simulink model "Plant"  (R2018b)
settings: configuration reference "plant_config" (kept outside this file)
values from neighbouring files (symbols this model uses):
  PLANT_EXPORT = Simulink.Parameter(PLANT_EXPORT_VALUE)    [plant_model_init.m]
  PLANT_PARAM = Simulink.Parameter(PLANT_PARAM_VALUE)    [plant_model_init.m]
undefined symbols (not defined in the file or in its folder): acc_x, acc_x_O, acc_y, acc_y_O, acc_z, acc_z_O, alt, alt_0, day, DiscIntNeverNeededParam, fixType, flags, ground_force, gSpeed, gyr_x, gyr_y, gyr_z, h_R, hAcc, heading, headingAcc, height, hMSL, hour, iTOW, lat, lon, M_BO, M_OB, mag_x, mag_y, mag_z, month, nano, numSV, pDOP, phi, PLANT_CONST, plant_model, pressure, prop_vel, psi, quat, reserved1, reserved2, rot_x_B, rot_y_B, rot_z_B, sAcc, sec, Sensor_Model, tAcc, temperature, temprature, theta, timestamp, vAcc, valid, vel_x_O, vel_y_O ... (+7)
libraries: FMT_Model_Lib x22, simulink x12, dspsrcs4 x6, aerolibatmos2 x1
(part 2 of 2)

== system Plant/Sensor_Model/Sensor_MAG/Magnetometer ==
  States : Inport
  Enable_Errors : Inport  Port=2
  Bus_Constructor : Subsystem
  Physical_Model : Subsystem
  Sensor_Model : Subsystem
  Mag_Raw : Outport
  wires:
  Bus_Constructor/1(Mag_Raw) -> Mag_Raw/1
  Sensor_Model/1(y) -> Bus_Constructor/1(Output)
  States/1 -> Physical_Model/1(States)
  Physical_Model/1(mag_B_gauss) -> Sensor_Model/2(u)
  Enable_Errors/1 -> Sensor_Model/1(Enable_Errors)

== system Plant/Actuators/Motors/ESCs/Rotor_Delay ==
  in : Inport
  Discrete-Time Integrator : DiscreteIntegrator  gainval=K  SampleTime=-1  ICPrevOutput=DiscIntNeverNeededParam  ICPrevScaledInput=DiscIntNeverNeededParam
  Gain : Gain  Gain=1/T
  Subtract : Sum  Inputs=+-
  out : Outport
  wires:
  in/1 -> Subtract/1
  Subtract/1 -> Gain/1
  Gain/1 -> Discrete-Time Integrator/1
  Discrete-Time Integrator/1 -> Subtract/2, out/1

== system Plant/Actuators/Motors/ESCs/Rotor_Speed ==
  u0 : Inport
  Add : Sum
  Compare To Constant : simulink/Logic and Bit Operations/Compare To Constant  relop=>  const=0.1  OutDataTypeStr=boolean
  Constant1 : Constant  Value=p  OutDataTypeStr=single
  Gain1 : Gain  Gain=k  OutDataTypeStr=Inherit: Same as input
  Multiply : Product
  Saturation1 : Saturate  UpperLimit=9999999  LowerLimit=0
  omega_B_radPs : Outport
  wires:
  Multiply/1 -> Saturation1/1
  Gain1/1 -> Add/1
  Saturation1/1 -> omega_B_radPs/1
  u0/1 -> Compare To Constant/1, Gain1/1
  Constant1/1 -> Add/2
  Compare To Constant/1 -> Multiply/1
  Add/1 -> Multiply/2

== system Plant/Actuators/Motors/Force/Rotor_Thrust ==
  rotor_speed_radPs : Inport
  Multiply : Product  OutDataTypeStr=Inherit: Same as first input
  Square : Math  Operator=square  SaturateOnIntegerOverflow=on
  cT : Constant  Value=cT
  thrust_B_N : Outport
  wires:
  rotor_speed_radPs/1 -> Square/1
  Square/1 -> Multiply/1
  cT/1 -> Multiply/2
  Multiply/1 -> thrust_B_N/1

== system Plant/Actuators/Motors/Torque/Gyroscopic_Torque ==
  rotor_speed_radPs : Inport
  omega_B_radPs : Inport  Port=2
  Add : Sum  Inputs=--++
  Constant : Constant  Value=[0;0;Im]  OutDataTypeStr=single
  Cross Product : FMT_Model_Lib/Math/Cross Product
      settings: SourceProductName=FMT Toolbox
  Demux : Demux
  Multiply : Product
  gyroscopic_torque : Outport
  wires:
  Demux/1 -> Add/1
  Constant/1 -> Cross Product/1
  Demux/4 -> Add/4
  Add/1 -> Multiply/1
  Demux/3 -> Add/3
  Demux/2 -> Add/2
  omega_B_radPs/1 -> Multiply/2
  Multiply/1 -> Cross Product/2
  Cross Product/1 -> gyroscopic_torque/1
  rotor_speed_radPs/1 -> Demux/1

== system Plant/Actuators/Motors/Torque/Rotor_Torque ==
  rotor_speed_radPs : Inport
  Multiply : Product  Multiplication=Matrix(*)
  Square : Math  Operator=square  SaturateOnIntegerOverflow=on
  X_Frame_CM : Constant  Value=[-L*cT,L*cT,L*cT,-L*cT;L*cT,-L*cT,L*cT,-L*cT;cQ,cQ,-cQ,-cQ]  OutDataTypeStr=single
  rotor_torque : Outport
  wires:
  X_Frame_CM/1 -> Multiply/1
  Square/1 -> Multiply/2
  Multiply/1 -> rotor_torque/1
  rotor_speed_radPs/1 -> Square/1

== system Plant/Kinematic_Equation/Attitude_Dynamic/Quaternuin_Update/Quaternion_Update_Maxtrix ==
  omega_B_radPs : Inport
  Constant{,1..3} (4 alike) : Constant  Value=0  OutDataTypeStr=single
  Demux : Demux  Outputs=3
  Gain{1..4,6..7} (6 alike) : Gain  Gain=-1  OutDataTypeStr=Inherit: Same as input
  Matrix Concatenate{,1..3} (4 alike) : Concatenate  NumInputs=4
  Matrix Concatenate4 : Concatenate  NumInputs=4  Mode=Multidimensional array  ConcatenateDimension=2
  W : Outport
  wires:
  Gain1/1 -> Matrix Concatenate1/1
  Gain7/1 -> Matrix Concatenate3/2
  Matrix Concatenate2/1 -> Matrix Concatenate4/3  "col3"
  Constant2/1 -> Matrix Concatenate2/3
  Matrix Concatenate4/1 -> W/1
  Demux/1 -> Matrix Concatenate/2, Gain1/1, Gain4/1, Matrix Concatenate3/3  "w1"
  Matrix Concatenate/1 -> Matrix Concatenate4/1  "col1"
  Matrix Concatenate1/1 -> Matrix Concatenate4/2  "col2"
  Constant3/1 -> Matrix Concatenate3/4
  Gain6/1 -> Matrix Concatenate3/1
  Constant1/1 -> Matrix Concatenate1/2
  Matrix Concatenate3/1 -> Matrix Concatenate4/4  "col4"
  Demux/2 -> Matrix Concatenate1/4, Gain3/1, Gain7/1, Matrix Concatenate/3  "w2"
  Constant/1 -> Matrix Concatenate/1
  Gain3/1 -> Matrix Concatenate2/1
  Demux/3 -> Gain2/1, Matrix Concatenate2/2, Gain6/1, Matrix Concatenate/4  "w3"
  Gain2/1 -> Matrix Concatenate1/3
  omega_B_radPs/1 -> Demux/1
  Gain4/1 -> Matrix Concatenate2/4

== system Plant/Sensor_Model/Sensor_Barometer/Barometer/Physical_Model ==
  States : Inport
  Bus Selector1 : BusSelector  OutputSignals=Plant_States.alt
  Data Type Conversion : DataTypeConversion  OutDataTypeStr=single
  ISA Atmosphere Model : aerolibatmos2/ISA Atmosphere Model  custom=off  g=9.80665  gamma=1.4  R=287.0531  L=0.0065  h_trop=11000  h_strat=20000  rho0=1.225  P0=101325  T0=288.15  h0=0
      settings: SourceProductName=Aerospace Blockset
  Terminator : Terminator
  Terminator1 : Terminator
  Pressure_Pa : Outport
  Temperature_K : Outport  Port=2
  wires:
  States/1 -> Bus Selector1/1
  ISA Atmosphere Model/1 -> Temperature_K/1
  ISA Atmosphere Model/2 -> Terminator1/1
  ISA Atmosphere Model/4 -> Terminator/1
  Bus Selector1/1 -> Data Type Conversion/1  "<alt>"
  ISA Atmosphere Model/3 -> Pressure_Pa/1
  Data Type Conversion/1 -> ISA Atmosphere Model/1

== system Plant/Sensor_Model/Sensor_Barometer/Barometer/Sensor_Model ==
  Enable_Errors : Inport
  u : Inport  Port=2
  Add : Sum  InputSameDT=on  OutDataTypeStr=Inherit: Same as first input
  Saturation : Saturate  UpperLimit=Sensor_Model.Baro.Upper_limit  LowerLimit=Sensor_Model.Baro.Lower_limit  OutDataTypeStr=single
  Sensor_Error : Subsystem
  Sensor_Noise : Subsystem
  Switch : Switch  Criteria=u2 > Threshold
  y : Outport
  wires:
  Switch/1 -> y/1
  Saturation/1 -> Add/1
  Sensor_Error/1(y) -> Saturation/1
  Enable_Errors/1 -> Switch/2
  u/1 -> Switch/3, Sensor_Error/1(u)
  Add/1 -> Switch/1
  Sensor_Noise/1(noise) -> Add/2

== system Plant/Sensor_Model/Sensor_GPS/Bus_Constructor/GroundSpeed ==
  u_O_mPs : Inport
  v_O_mPs : Inport  Port=2
  Add : Sum
  Math Function : Math  Operator=square  SaturateOnIntegerOverflow=on
  Math Function1 : Math  Operator=square  SaturateOnIntegerOverflow=on
  Saturation : Saturate  UpperLimit=inf  LowerLimit=0
  Sqrt : Sqrt  SaturateOnIntegerOverflow=on
  gSpeed_mPs : Outport
  wires:
  Sqrt/1 -> gSpeed_mPs/1
  Math Function/1 -> Add/1
  Math Function1/1 -> Add/2
  Saturation/1 -> Sqrt/1
  Add/1 -> Saturation/1
  u_O_mPs/1 -> Math Function/1
  v_O_mPs/1 -> Math Function1/1

== system Plant/Sensor_Model/Sensor_GPS/Bus_Constructor/WGS84_Position ==
  pos_WGS84 : Inport
  Demux1 : Demux  Outputs=3
  Signal Conversion : SignalConversion  OverrideOpt=off
  Signal Conversion1 : SignalConversion  OverrideOpt=off
  Signal Conversion2 : SignalConversion  OverrideOpt=off
  lon : Outport
  lat : Outport  Port=2
  height : Outport  Port=3
  wires:
  Demux1/3 -> Signal Conversion2/1  "POS_h_WGS84"
  Signal Conversion/1 -> lon/1
  Demux1/1 -> Signal Conversion/1  "POS_lon_WGS84"
  pos_WGS84/1 -> Demux1/1
  Demux1/2 -> Signal Conversion1/1  "POS_lat_WGS84"
  Signal Conversion1/1 -> lat/1
  Signal Conversion2/1 -> height/1

== system Plant/Sensor_Model/Sensor_GPS/GPS/Bus_Constructor ==
  WGS84_pos_meas : Inport
  vel_O_meas : Inport  Port=2
  numSV : Inport  Port=3
  fixType : Inport  Port=4
  h_Acc_m : Inport  Port=5
  v_Acc_m : Inport  Port=6
  s_Acc_mDs : Inport  Port=7
  Bus Creator : BusCreator  Inputs=7
  GPS_Raw : Outport
  wires:
  WGS84_pos_meas/1 -> Bus Creator/1  "WGS84_pos"
  vel_O_meas/1 -> Bus Creator/2  "vel_O"
  numSV/1 -> Bus Creator/3  "numSV"
  fixType/1 -> Bus Creator/4  "fixType"
  h_Acc_m/1 -> Bus Creator/5  "hAcc"
  v_Acc_m/1 -> Bus Creator/6  "vAcc"
  s_Acc_mDs/1 -> Bus Creator/7  "sAcc"
  Bus Creator/1 -> GPS_Raw/1

== system Plant/Sensor_Model/Sensor_GPS/GPS/Physical_Model ==
  note: Transfer Delay
  States : Inport
  Bus Selector : BusSelector  OutputSignals=Plant_States.lon,Plant_States.lat,Plant_States.alt
  Bus Selector1 : BusSelector  OutputSignals=Plant_States.vel_x_O,Plant_States.vel_y_O,Plant_States.vel_z_O
  Delay : Delay  DelayLength=150/(PLANT_CONST.dt*1e3)
  Delay1 : Delay  DelayLength=100/(PLANT_CONST.dt*1e3)
  Vector Concatenate : Concatenate  NumInputs=3  Mode=Multidimensional array
  Vector Concatenate1 : Concatenate  NumInputs=3  Mode=Multidimensional array
  WGS84_pos_rad : Outport  Unit=rad/s
  vel_O_mPs : Outport  Port=2  Unit=m/s  PortDimensions=[3 1]
  wires:
  Bus Selector/3 -> Vector Concatenate/3  "<alt>"
  Bus Selector/2 -> Vector Concatenate/2  "<lat>"
  Bus Selector/1 -> Vector Concatenate/1  "<lon>"
  Vector Concatenate/1 -> Delay/1
  Bus Selector1/2 -> Vector Concatenate1/2  "<vel_y_O>"
  Bus Selector1/3 -> Vector Concatenate1/3  "<vel_z_O>"
  States/1 -> Bus Selector1/1, Bus Selector/1
  Vector Concatenate1/1 -> Delay1/1
  Bus Selector1/1 -> Vector Concatenate1/1  "<vel_x_O>"
  Delay/1 -> WGS84_pos_rad/1
  Delay1/1 -> vel_O_mPs/1

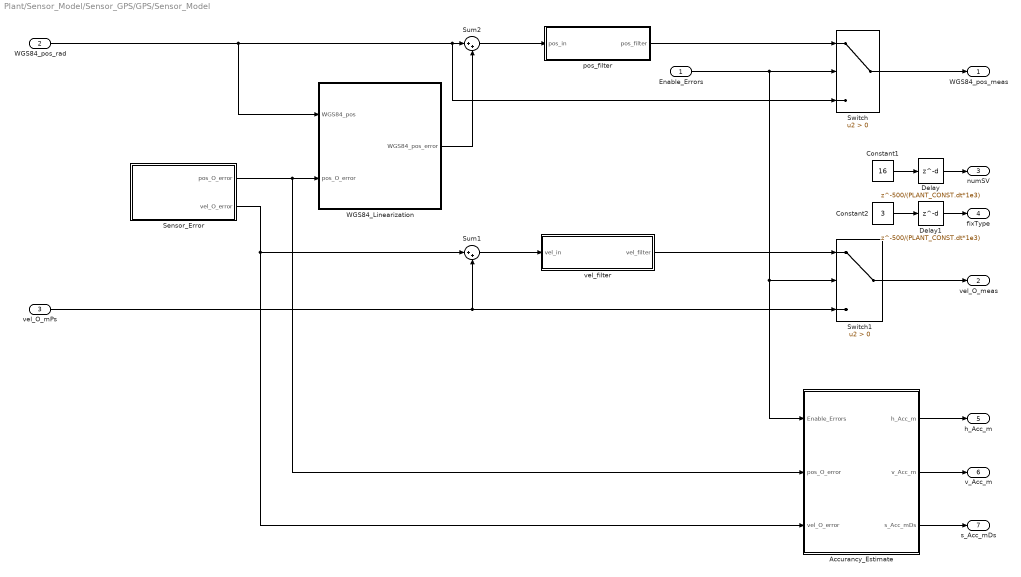
== system Plant/Sensor_Model/Sensor_GPS/GPS/Sensor_Model ==
  Enable_Errors : Inport
  WGS84_pos_rad : Inport  Port=2
  vel_O_mPs : Inport  Port=3
  Accurancy_Estimate : Subsystem
  Constant1 : Constant  Value=16  OutDataTypeStr=Inherit: Inherit via back propagation
  Constant2 : Constant  Value=3  OutDataTypeStr=Inherit: Inherit via back propagation
  Delay : Delay  DelayLength=500/(PLANT_CONST.dt*1e3)
  Delay1 : Delay  DelayLength=500/(PLANT_CONST.dt*1e3)
  Sensor_Error : Subsystem
  Sum1 : Sum  Inputs=|++
  Sum2 : Sum  Inputs=|++
  Switch : Switch  Criteria=u2 > Threshold
  Switch1 : Switch  Criteria=u2 > Threshold
  WGS84_Linearization : Subsystem
  pos_filter : Subsystem
  vel_filter : Subsystem
  WGS84_pos_meas : Outport
  vel_O_meas : Outport  Port=2
  numSV : Outport  Port=3
  fixType : Outport  Port=4
  h_Acc_m : Outport  Port=5
  v_Acc_m : Outport  Port=6
  s_Acc_mDs : Outport  Port=7
  wires:
  Constant2/1 -> Delay1/1
  Constant1/1 -> Delay/1
  Switch/1 -> WGS84_pos_meas/1
  Switch1/1 -> vel_O_meas/1
  Sum2/1 -> pos_filter/1(pos_in)
  Sensor_Error/1(pos_O_error) -> Accurancy_Estimate/2(pos_O_error), WGS84_Linearization/2(pos_O_error)
  Sum1/1 -> vel_filter/1(vel_in)
  Sensor_Error/2(vel_O_error) -> Accurancy_Estimate/3(vel_O_error), Sum1/1
  WGS84_Linearization/1(WGS84_pos_error) -> Sum2/2
  Accurancy_Estimate/1(h_Acc_m) -> h_Acc_m/1
  Accurancy_Estimate/3(s_Acc_mDs) -> s_Acc_mDs/1
  Accurancy_Estimate/2(v_Acc_m) -> v_Acc_m/1
  pos_filter/1(pos_filter) -> Switch/1
  WGS84_pos_rad/1 -> Switch/3, Sum2/1, WGS84_Linearization/1(WGS84_pos)
  vel_O_mPs/1 -> Switch1/3, Sum1/2
  vel_filter/1(vel_filter) -> Switch1/1
  Enable_Errors/1 -> Switch/2, Accurancy_Estimate/1(Enable_Errors), Switch1/2
  Delay/1 -> numSV/1
  Delay1/1 -> fixType/1

== system Plant/Sensor_Model/Sensor_IMU/Accelerometer/Bus_Constructor ==
  Output : Inport
  Bus Creator : BusCreator  Inputs=3
  Demux : Demux  Outputs=3
  Acc_Raw : Outport
  wires:
  Demux/2 -> Bus Creator/2  "Acc_y_mPs2"
  Demux/3 -> Bus Creator/3  "Acc_z_mPs2"
  Demux/1 -> Bus Creator/1  "Acc_x_mPs2"
  Bus Creator/1 -> Acc_Raw/1
  Output/1 -> Demux/1

== system Plant/Sensor_Model/Sensor_IMU/Accelerometer/Physical_Model ==
  States : Inport
  Enable_Errors : Inport  Port=2
  Sum : Sum  Inputs=|++
  Switch : Switch  Criteria=u2 > Threshold  OutDataTypeStr=single
  Vibration_Model : Subsystem  TreatAsAtomicUnit=on  mask{gain=Sensor_Model.Acc.Vibration.Gain}
      mask prompts: gain "Vibration gain"
      mask help: propeller vibration model
      settings: RTWSystemCode=Inline
  prop_vel : Subsystem
  specific_force : Subsystem
  sfor_B_mPs2 : Outport  Unit=m/s^2
  wires:
  States/1 -> specific_force/1(States), prop_vel/1(States)
  Switch/1 -> sfor_B_mPs2/1
  prop_vel/1(omega_radDs) -> Vibration_Model/1(prop_rot_radPs)
  specific_force/1(sfor_B_mPs2) -> Sum/2, Switch/3
  Enable_Errors/1 -> Switch/2
  Vibration_Model/1(vibration) -> Sum/1
  Sum/1 -> Switch/1

== system Plant/Sensor_Model/Sensor_IMU/Accelerometer/Sensor_Model ==
  Enable_Errors : Inport
  u : Inport  Port=2
  First Order LPF : FMT_Model_Lib/Filter/First Order LPF  fc=Sensor_Model.Acc.Cutoff_frequency_Hz
      settings: SourceProductName=FMT Toolbox
  Saturation : Saturate  UpperLimit=Sensor_Model.Acc.Upper_limit  LowerLimit=Sensor_Model.Acc.Lower_limit
  Sensor_Error : Subsystem
  Sensor_Noise : Subsystem
  Sum : Sum  Inputs=|++
  Switch : Switch  Criteria=u2 > Threshold
  y : Outport
  wires:
  Switch/1 -> y/1
  Saturation/1 -> Sum/1
  First Order LPF/1 -> Saturation/1
  Sensor_Error/1(y) -> First Order LPF/1
  Sensor_Noise/1(noise) -> Sum/2
  Enable_Errors/1 -> Switch/2
  u/1 -> Switch/3, Sensor_Error/1(u)
  Sum/1 -> Switch/1

== system Plant/Sensor_Model/Sensor_IMU/Gyroscope/Bus_Constructor ==
  Output : Inport
  Bus Creator : BusCreator  Inputs=3
  Demux : Demux  Outputs=3
  Gyro_Raw : Outport
  wires:
  Demux/1 -> Bus Creator/1  "Gyro_x_radPs"
  Demux/2 -> Bus Creator/2  "Gyro_y_radPs"
  Demux/3 -> Bus Creator/3  "Gyro_z_radPs"
  Bus Creator/1 -> Gyro_Raw/1
  Output/1 -> Demux/1

== system Plant/Sensor_Model/Sensor_IMU/Gyroscope/Physical_Model ==
  States : Inport
  Enable_Errors : Inport  Port=2
  Sum : Sum  Inputs=|++
  Switch : Switch  Criteria=u2 > Threshold
  Vibration_Model : Subsystem  TreatAsAtomicUnit=on  mask{gain=Sensor_Model.Gyro.Vibration.Gain}
      mask prompts: gain "Vibration gain"
      mask help: propeller vibration model
      settings: RTWSystemCode=Inline
  prop_vel : Subsystem
  rotation_speed : Subsystem
  gyr_B_radDs : Outport  Unit=rad/s
  wires:
  States/1 -> rotation_speed/1(States), prop_vel/1(States)
  Switch/1 -> gyr_B_radDs/1
  prop_vel/1(omega_radPs) -> Vibration_Model/1(prop_rot_radPs)
  rotation_speed/1(rot_radPs) -> Sum/2, Switch/3
  Enable_Errors/1 -> Switch/2
  Vibration_Model/1(vibration) -> Sum/1
  Sum/1 -> Switch/1

== system Plant/Sensor_Model/Sensor_IMU/Gyroscope/Sensor_Model ==
  Enable_Errors : Inport
  u : Inport  Port=2
  First Order LPF : FMT_Model_Lib/Filter/First Order LPF  fc=Sensor_Model.Gyro.Cutoff_frequency_Hz
      settings: SourceProductName=FMT Toolbox
  Saturation : Saturate  UpperLimit=Sensor_Model.Gyro.Range  LowerLimit=-Sensor_Model.Gyro.Range
  Sensor_Error : Subsystem
  Sensor_Noise : Subsystem
  Sum : Sum  Inputs=|++
  Switch : Switch  Criteria=u2 > Threshold
  y : Outport
  wires:
  Switch/1 -> y/1
  Saturation/1 -> Sum/1
  First Order LPF/1 -> Saturation/1
  Sensor_Error/1(y) -> First Order LPF/1
  Sensor_Noise/1(noise) -> Sum/2
  Enable_Errors/1 -> Switch/2
  u/1 -> Switch/3, Sensor_Error/1(u)
  Sum/1 -> Switch/1

== system Plant/Sensor_Model/Sensor_MAG/Magnetometer/Bus_Constructor ==
  Output : Inport
  Bus Creator : BusCreator  Inputs=3
  Demux : Demux  Outputs=3
  Mag_Raw : Outport
  wires:
  Demux/2 -> Bus Creator/2  "Mag_y_gauss"
  Demux/1 -> Bus Creator/1  "Mag_x_gauss"
  Bus Creator/1 -> Mag_Raw/1
  Demux/3 -> Bus Creator/3  "Mag_z_gauss"
  Output/1 -> Demux/1

== system Plant/Sensor_Model/Sensor_MAG/Magnetometer/Physical_Model ==
  States : Inport
  Bus Selector : BusSelector  OutputSignals=Plant_States.lat,Plant_States.lon
  Bus Selector1 : BusSelector  OutputSignals=Extended_States.M_BO
  Product : Product  Multiplication=Matrix(*)  RndMeth=Zero  InputSameDT=on  OutDataTypeStr=Inherit: Same as first input
  WMM_LUT : Subsystem  mask{wmm_magnitude=Sensor_Model.Mag.WMM_Mag, wmm_declination=Sensor_Model.Mag.WMM_Dec, wmm_inclination=Sensor_Model.Mag.WMM_Inc, resolution=10}
      mask prompts: wmm_magnitude "WMM Magnitude Lookup Table"; wmm_declination "WMM Declination Lookup Table"; wmm_inclination "WMM Inclination Lookup Table"; resolution "Resolution (deg)"
  magnetic_field : Subsystem
  mag_B_gauss : Outport  Unit=T  PortDimensions=[3 1]
  wires:
  States/1 -> Bus Selector1/1, Bus Selector/1
  Bus Selector/2 -> WMM_LUT/2(lon_rad)  "<lon>"
  Bus Selector/1 -> WMM_LUT/1(lat_rad)  "<lat>"
  Bus Selector1/1 -> Product/1  "<M_BO>"
  Product/1 -> mag_B_gauss/1
  magnetic_field/1(mag_O_gauss) -> Product/2
  WMM_LUT/1(magnitude_uT) -> magnetic_field/1(magnitude_uT)
  WMM_LUT/2(declination_deg) -> magnetic_field/2(declination_deg)
  WMM_LUT/3(inclination_deg) -> magnetic_field/3(inclination_deg)

== system Plant/Sensor_Model/Sensor_MAG/Magnetometer/Sensor_Model ==
  Enable_Errors : Inport
  u : Inport  Port=2
  Add : Sum  InputSameDT=on  OutDataTypeStr=Inherit: Same as first input
  Saturation : Saturate  UpperLimit=Sensor_Model.Mag.Upper_limit  LowerLimit=Sensor_Model.Mag.Lower_limit
  Sensor_Error : Subsystem
  Sensor_Noise : Subsystem
  Switch : Switch  Criteria=u2 > Threshold
  y : Outport
  wires:
  Switch/1 -> y/1
  Saturation/1 -> Add/1
  Sensor_Error/1(y) -> Saturation/1
  Sensor_Noise/1(noise) -> Add/2
  Enable_Errors/1 -> Switch/2
  u/1 -> Switch/3, Sensor_Error/1(u)
  Add/1 -> Switch/1

== system Plant/Sensor_Model/Sensor_Barometer/Barometer/Sensor_Model/Sensor_Error ==
  u : Inport
  Constant3 : Constant  Value=Sensor_Model.Baro.Bias  VectorParams1D=off  OutDataTypeStr=single
  Sum : Sum  Inputs=|++  InputSameDT=on  OutDataTypeStr=Inherit: Same as first input
  y : Outport
  wires:
  Sum/1 -> y/1
  u/1 -> Sum/1
  Constant3/1 -> Sum/2

== system Plant/Sensor_Model/Sensor_Barometer/Barometer/Sensor_Model/Sensor_Noise ==
  Random Source : dspsrcs4/Random Source  SrcType=Gaussian  NormMethod=Ziggurat  CltLength=12  MinVal=0  MaxVal=1  MeanVal=0  VarVal=Sensor_Model.Baro.Variance  RepMode=Repeatable  rawSeed=1  IsInherit=off  SampMode=Discrete  SampTime=-1  SampFrame=1  DataType=Single  OutComplex=Real  OutputFrames=off
  noise : Outport
  wires:
  Random Source/1 -> noise/1

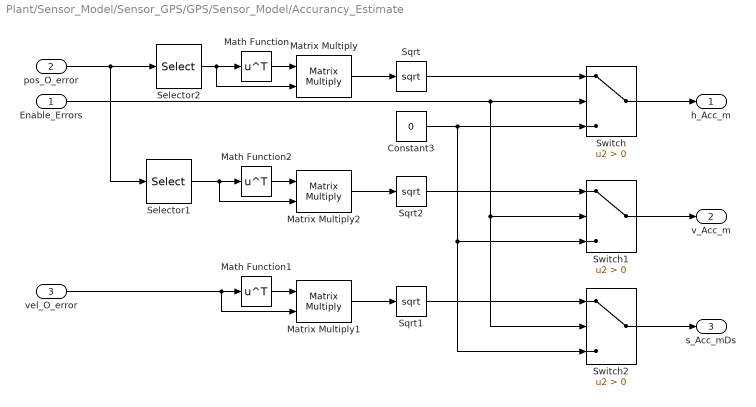
== system Plant/Sensor_Model/Sensor_GPS/GPS/Sensor_Model/Accurancy_Estimate ==
  Enable_Errors : Inport
  pos_O_error : Inport  Port=2
  vel_O_error : Inport  Port=3
  Constant3 : Constant  Value=0
  Math Function : Math  Operator=transpose  SaturateOnIntegerOverflow=on
  Math Function1 : Math  Operator=transpose  SaturateOnIntegerOverflow=on
  Math Function2 : Math  Operator=transpose  SaturateOnIntegerOverflow=on
  Matrix Multiply : Product  Multiplication=Matrix(*)
  Matrix Multiply1 : Product  Multiplication=Matrix(*)
  Matrix Multiply2 : Product  Multiplication=Matrix(*)
  Selector1 : Selector  InputPortWidth=3  IndexOptions=Index vector (dialog)  Indices=3  OutputSizes=1
  Selector2 : Selector  InputPortWidth=3  IndexOptions=Index vector (dialog)  Indices=[1 2]  OutputSizes=1
  Sqrt : Sqrt  OutputSignalType=real  SaturateOnIntegerOverflow=on
  Sqrt1 : Sqrt  OutputSignalType=real  SaturateOnIntegerOverflow=on
  Sqrt2 : Sqrt  OutputSignalType=real  SaturateOnIntegerOverflow=on
  Switch : Switch  Criteria=u2 > Threshold
  Switch1 : Switch  Criteria=u2 > Threshold
  Switch2 : Switch  Criteria=u2 > Threshold
  h_Acc_m : Outport
  v_Acc_m : Outport  Port=2
  s_Acc_mDs : Outport  Port=3
  wires:
  Switch/1 -> h_Acc_m/1
  pos_O_error/1 -> Selector1/1, Selector2/1
  Switch1/1 -> v_Acc_m/1
  Selector1/1 -> Math Function2/1, Matrix Multiply2/2
  Switch2/1 -> s_Acc_mDs/1
  Math Function1/1 -> Matrix Multiply1/1
  Math Function2/1 -> Matrix Multiply2/1
  Math Function/1 -> Matrix Multiply/1
  Selector2/1 -> Matrix Multiply/2, Math Function/1
  Matrix Multiply1/1 -> Sqrt1/1
  Matrix Multiply/1 -> Sqrt/1
  Matrix Multiply2/1 -> Sqrt2/1
  vel_O_error/1 -> Matrix Multiply1/2, Math Function1/1
  Sqrt/1 -> Switch/1
  Sqrt2/1 -> Switch1/1
  Enable_Errors/1 -> Switch2/2, Switch1/2, Switch/2
  Sqrt1/1 -> Switch2/1
  Constant3/1 -> Switch2/3, Switch1/3, Switch/3

== system Plant/Sensor_Model/Sensor_GPS/GPS/Sensor_Model/Sensor_Error ==
  Random Source : dspsrcs4/Random Source  SrcType=Gaussian  NormMethod=Ziggurat  CltLength=12  MinVal=0  MaxVal=1  MeanVal=0  VarVal=[0.2;0.2;0.4].^2  RepMode=Repeatable  rawSeed=1  IsInherit=off  SampMode=Discrete  SampTime=-1  SampFrame=1  DataType=Single  OutComplex=Real  OutputFrames=off
  Random Source1 : dspsrcs4/Random Source  SrcType=Gaussian  NormMethod=Ziggurat  CltLength=12  MinVal=0  MaxVal=1  MeanVal=0  VarVal=[0.01;0.01;0.01].^2  RepMode=Repeatable  rawSeed=1  IsInherit=off  SampMode=Discrete  SampTime=-1  SampFrame=1  DataType=Single  OutComplex=Real  OutputFrames=off
  pos_O_error : Outport
  vel_O_error : Outport  Port=2
  wires:
  Random Source/1 -> pos_O_error/1
  Random Source1/1 -> vel_O_error/1

== system Plant/Sensor_Model/Sensor_GPS/GPS/Sensor_Model/WGS84_Linearization ==
  WGS84_pos : Inport
  pos_O_error : Inport  Port=2
  Demux2 : Demux  Outputs=3
  Divide2 : Product  Inputs=/*
  LAT2FLAT Curve : FMT_Model_Lib/Transformation/LAT2FLAT Curve
      settings: SourceProductName=FMT Toolbox
  Terminator1 : Terminator
  Terminator2 : Terminator
  Vector Concatenate2 : Concatenate  NumInputs=3  Mode=Multidimensional array
  constant1 : Constant  Value=-1
  WGS84_pos_error : Outport
  wires:
  WGS84_pos/1 -> Demux2/1
  Demux2/1 -> LAT2FLAT Curve/1
  LAT2FLAT Curve/2 -> Vector Concatenate2/2
  pos_O_error/1 -> Divide2/2
  Vector Concatenate2/1 -> Divide2/1
  LAT2FLAT Curve/1 -> Vector Concatenate2/1
  Demux2/2 -> Terminator2/1
  Demux2/3 -> Terminator1/1
  constant1/1 -> Vector Concatenate2/3
  Divide2/1 -> WGS84_pos_error/1

== system Plant/Sensor_Model/Sensor_GPS/GPS/Sensor_Model/pos_filter ==
  pos_in : Inport
  Discrete FIR Filter : DiscreteFir
  pos_filter : Outport
  wires:
  Discrete FIR Filter/1 -> pos_filter/1
  pos_in/1 -> Discrete FIR Filter/1

== system Plant/Sensor_Model/Sensor_GPS/GPS/Sensor_Model/vel_filter ==
  vel_in : Inport
  Discrete FIR Filter : DiscreteFir
  vel_filter : Outport
  wires:
  Discrete FIR Filter/1 -> vel_filter/1
  vel_in/1 -> Discrete FIR Filter/1

== system Plant/Sensor_Model/Sensor_IMU/Accelerometer/Physical_Model/Vibration_Model ==
  prop_rot_radPs : Inport  PortDimensions=[4,1]
  Compare To Constant1 : simulink/Logic and Bit Operations/Compare To Constant  relop=>  const=4*pi  OutDataTypeStr=boolean
  Discrete-Time Integrator : DiscreteIntegrator  InitialCondition=zeros(4,1)  SampleTime=-1  ICPrevOutput=DiscIntNeverNeededParam  ICPrevScaledInput=DiscIntNeverNeededParam
  Divide : Product  Inputs=*/
  Gain2 : Gain  Gain=0.5
  Gain4 : Gain  Gain=gain
  Product1 : Product  RndMeth=Zero
  Product2 : Product  RndMeth=Zero
  Reshape : Reshape  OutputDimensionality=Column vector (2-D)
  Saturation : Saturate  UpperLimit=8  LowerLimit=4
  Sum : Sum  Inputs=++|
  Sum of Elements : Sum  Inputs=+
  Sum of Elements1 : Sum  Inputs=+
  Sum of Elements2 : Sum  Inputs=+  CollapseMode=Specified dimension
  Trigonometric Function1 : Trigonometry  Operator=cos
  Trigonometric Function2 : Trigonometry
  Vector Concatenate : Concatenate  NumInputs=3  Mode=Multidimensional array
  vib_frequency : Subsystem
  vibration : Outport
  wires:
  Sum of Elements2/1 -> Saturation/1
  Saturation/1 -> Divide/2
  Divide/1 -> Gain4/1
  Compare To Constant1/1 -> Sum of Elements2/1
  Vector Concatenate/1 -> Divide/1
  Trigonometric Function1/1 -> Product1/1
  Trigonometric Function2/1 -> Product2/1
  Gain2/1 -> Vector Concatenate/3
  Sum/1 -> Gain2/1
  Sum of Elements1/1 -> Sum/2, Vector Concatenate/2
  Discrete-Time Integrator/1 -> Trigonometric Function1/1, Trigonometric Function2/1
  Sum of Elements/1 -> Vector Concatenate/1, Sum/1
  Reshape/1 -> vibration/1
  Gain4/1 -> Reshape/1
  prop_rot_radPs/1 -> Compare To Constant1/1, Discrete-Time Integrator/1, vib_frequency/1(prop_rot_radPs)
  vib_frequency/1(y) -> Product2/2, Product1/2
  Product2/1 -> Sum of Elements/1
  Product1/1 -> Sum of Elements1/1

== system Plant/Sensor_Model/Sensor_IMU/Accelerometer/Physical_Model/prop_vel ==
  States : Inport
  Bus Selector2 : BusSelector  OutputSignals=Extended_States.prop_vel
  Selector : Selector  InputPortWidth=8  IndexOptions=Index vector (dialog)  Indices=[1:4]  OutputSizes=1
  omega_radDs : Outport
  wires:
  States/1 -> Bus Selector2/1
  Bus Selector2/1 -> Selector/1  "<prop_vel>"
  Selector/1 -> omega_radDs/1

== system Plant/Sensor_Model/Sensor_IMU/Accelerometer/Physical_Model/specific_force ==
  States : Inport
  Bus Selector : BusSelector  OutputSignals=Plant_States.acc_x_O,Plant_States.acc_y_O,Plant_States.acc_z_O
  Bus Selector1 : BusSelector  OutputSignals=Extended_States.M_BO
  Gravity : Constant  Value=[0;0;Sensor_Model.g]  OutDataTypeStr=single
  Product1 : Product  Multiplication=Matrix(*)  RndMeth=Zero  InputSameDT=on  OutDataTypeStr=Inherit: Same as first input
  Sum : Sum  Inputs=|+-  InputSameDT=on  OutDataTypeStr=Inherit: Same as first input
  Vector Concatenate1 : Concatenate  NumInputs=3  Mode=Multidimensional array
  sfor_B_mPs2 : Outport  Unit=m/s^2
  wires:
  States/1 -> Bus Selector1/1, Bus Selector/1
  Bus Selector/1 -> Vector Concatenate1/1  "<acc_x_O>"
  Bus Selector/2 -> Vector Concatenate1/2  "<acc_y_O>"
  Bus Selector/3 -> Vector Concatenate1/3  "<acc_z_O>"
  Product1/1 -> sfor_B_mPs2/1
  Bus Selector1/1 -> Product1/1  "<M_BO>"
  Vector Concatenate1/1 -> Sum/1
  Sum/1 -> Product1/2
  Gravity/1 -> Sum/2

== system Plant/Sensor_Model/Sensor_IMU/Accelerometer/Sensor_Model/Sensor_Error ==
  u : Inport
  Add : Sum  InputSameDT=on  OutDataTypeStr=Inherit: Same as first input
  Constant : Constant  Value=eye(3)  OutDataTypeStr=single
  Constant1 : Constant  Value=Sensor_Model.Acc.Scalefactor_Error  VectorParams1D=off  OutDataTypeStr=single
  Constant3 : Constant  Value=Sensor_Model.Acc.Bias  VectorParams1D=off  OutDataTypeStr=single
  Product : Product  Multiplication=Matrix(*)  RndMeth=Zero  InputSameDT=on  OutDataTypeStr=Inherit: Same as first input
  Sum : Sum  Inputs=|++  InputSameDT=on  OutDataTypeStr=Inherit: Same as first input
  y : Outport
  wires:
  Sum/1 -> y/1
  Add/1 -> Product/1
  u/1 -> Product/2
  Constant1/1 -> Add/2
  Constant/1 -> Add/1
  Product/1 -> Sum/1
  Constant3/1 -> Sum/2

== system Plant/Sensor_Model/Sensor_IMU/Accelerometer/Sensor_Model/Sensor_Noise ==
  Random Source : dspsrcs4/Random Source  SrcType=Gaussian  NormMethod=Ziggurat  CltLength=12  MinVal=0  MaxVal=1  MeanVal=0  VarVal=Sensor_Model.Acc.Variance  RepMode=Repeatable  rawSeed=1  IsInherit=off  SampMode=Discrete  SampTime=-1  SampFrame=1  DataType=Single  OutComplex=Real  OutputFrames=off
  noise : Outport
  wires:
  Random Source/1 -> noise/1

== system Plant/Sensor_Model/Sensor_IMU/Gyroscope/Physical_Model/Vibration_Model ==
  prop_rot_radPs : Inport  PortDimensions=[4,1]
  Compare To Constant1 : simulink/Logic and Bit Operations/Compare To Constant  relop=>  const=4*pi  OutDataTypeStr=boolean
  Discrete-Time Integrator : DiscreteIntegrator  InitialCondition=zeros(4,1)  SampleTime=-1  ICPrevOutput=DiscIntNeverNeededParam  ICPrevScaledInput=DiscIntNeverNeededParam
  Divide : Product  Inputs=*/
  Gain2 : Gain  Gain=0.5
  Gain4 : Gain  Gain=gain
  Product1 : Product  RndMeth=Zero
  Product2 : Product  RndMeth=Zero
  Reshape : Reshape  OutputDimensionality=Column vector (2-D)
  Saturation : Saturate  UpperLimit=8  LowerLimit=4
  Sum : Sum  Inputs=++|
  Sum of Elements : Sum  Inputs=+
  Sum of Elements1 : Sum  Inputs=+
  Sum of Elements2 : Sum  Inputs=+  CollapseMode=Specified dimension
  Trigonometric Function1 : Trigonometry  Operator=cos
  Trigonometric Function2 : Trigonometry
  Vector Concatenate : Concatenate  NumInputs=3  Mode=Multidimensional array
  vib_frequency : Subsystem
  vibration : Outport
  wires:
  Sum of Elements2/1 -> Saturation/1
  Saturation/1 -> Divide/2
  Divide/1 -> Gain4/1
  Compare To Constant1/1 -> Sum of Elements2/1
  Vector Concatenate/1 -> Divide/1
  Trigonometric Function1/1 -> Product1/1
  Trigonometric Function2/1 -> Product2/1
  Gain2/1 -> Vector Concatenate/3
  Sum/1 -> Gain2/1
  Sum of Elements1/1 -> Sum/2, Vector Concatenate/2
  Discrete-Time Integrator/1 -> Trigonometric Function1/1, Trigonometric Function2/1
  Sum of Elements/1 -> Vector Concatenate/1, Sum/1
  Reshape/1 -> vibration/1
  Gain4/1 -> Reshape/1
  prop_rot_radPs/1 -> Compare To Constant1/1, Discrete-Time Integrator/1, vib_frequency/1(prop_rot_radPs)
  vib_frequency/1(y) -> Product2/2, Product1/2
  Product2/1 -> Sum of Elements/1
  Product1/1 -> Sum of Elements1/1

== system Plant/Sensor_Model/Sensor_IMU/Gyroscope/Physical_Model/prop_vel ==
  States : Inport
  Bus Selector2 : BusSelector  OutputSignals=Extended_States.prop_vel
  Selector : Selector  InputPortWidth=8  IndexOptions=Index vector (dialog)  Indices=[1:4]  OutputSizes=1
  omega_radPs : Outport
  wires:
  Selector/1 -> omega_radPs/1
  States/1 -> Bus Selector2/1
  Bus Selector2/1 -> Selector/1  "<prop_vel>"

== system Plant/Sensor_Model/Sensor_IMU/Gyroscope/Physical_Model/rotation_speed ==
  States : Inport
  Bus Selector2 : BusSelector  OutputSignals=Plant_States.rot_x_B,Plant_States.rot_y_B,Plant_States.rot_z_B
  Vector Concatenate : Concatenate  NumInputs=3  Mode=Multidimensional array
  rot_radPs : Outport
  wires:
  Vector Concatenate/1 -> rot_radPs/1
  Bus Selector2/3 -> Vector Concatenate/3  "<rot_z_B>"
  Bus Selector2/1 -> Vector Concatenate/1  "<rot_x_B>"
  Bus Selector2/2 -> Vector Concatenate/2  "<rot_y_B>"
  States/1 -> Bus Selector2/1

== system Plant/Sensor_Model/Sensor_IMU/Gyroscope/Sensor_Model/Sensor_Error ==
  u : Inport
  Add : Sum  InputSameDT=on  OutDataTypeStr=Inherit: Same as first input
  Constant1 : Constant  Value=Sensor_Model.Gyro.Scalefactor_Error  VectorParams1D=off  OutDataTypeStr=single
  Constant2 : Constant  Value=eye(3)  OutDataTypeStr=single
  Constant3 : Constant  Value=Sensor_Model.Gyro.Bias  VectorParams1D=off  OutDataTypeStr=single
  Product : Product  Multiplication=Matrix(*)  RndMeth=Zero  InputSameDT=on  OutDataTypeStr=Inherit: Same as first input
  Sum : Sum  Inputs=|++  InputSameDT=on  OutDataTypeStr=Inherit: Same as first input
  y : Outport
  wires:
  Sum/1 -> y/1
  Product/1 -> Sum/1
  u/1 -> Product/2
  Add/1 -> Product/1
  Constant1/1 -> Add/2
  Constant2/1 -> Add/1
  Constant3/1 -> Sum/2

== system Plant/Sensor_Model/Sensor_IMU/Gyroscope/Sensor_Model/Sensor_Noise ==
  Random Source : dspsrcs4/Random Source  SrcType=Gaussian  NormMethod=Ziggurat  CltLength=12  MinVal=0  MaxVal=1  MeanVal=0  VarVal=Sensor_Model.Gyro.Variance  RepMode=Repeatable  rawSeed=1  IsInherit=off  SampMode=Discrete  SampTime=-1  SampFrame=1  DataType=Single  OutComplex=Real  OutputFrames=off
  noise : Outport
  wires:
  Random Source/1 -> noise/1

== system Plant/Sensor_Model/Sensor_MAG/Magnetometer/Physical_Model/WMM_LUT ==
  lat_rad : Inport
  lon_rad : Inport  Port=2
  Add : Sum
  Declination_Lookup_Table : LookupNDDirect  Table=wmm_declination  DiagnosticForOutOfRangeInput=Error
  Demux : Demux  Outputs=2
  Inclination_Lookup_Table : LookupNDDirect  Table=wmm_inclination  DiagnosticForOutOfRangeInput=Error
  Magnitude_Lookup_Table : LookupNDDirect  Table=wmm_magnitude  DiagnosticForOutOfRangeInput=Error
  Mux : Mux  Inputs=2
  Saturation1 : Saturate  UpperLimit=size(wmm_magnitude)-1  LowerLimit=0
  offset : Constant  Value=(size(wmm_magnitude)-1)/2  OutDataTypeStr=int32
  rad_to_index : Gain  Gain=180/pi/resolution  OutDataTypeStr=int32
  magnitude_uT : Outport
  declination_deg : Outport  Port=2
  inclination_deg : Outport  Port=3
  wires:
  Inclination_Lookup_Table/1 -> inclination_deg/1
  Declination_Lookup_Table/1 -> declination_deg/1
  Magnitude_Lookup_Table/1 -> magnitude_uT/1
  offset/1 -> Add/2
  Add/1 -> Saturation1/1
  rad_to_index/1 -> Add/1
  lat_rad/1 -> Mux/1
  lon_rad/1 -> Mux/2
  Mux/1 -> rad_to_index/1
  Saturation1/1 -> Demux/1
  Demux/1 -> Magnitude_Lookup_Table/1, Inclination_Lookup_Table/1, Declination_Lookup_Table/1
  Demux/2 -> Inclination_Lookup_Table/2, Magnitude_Lookup_Table/2, Declination_Lookup_Table/2

== system Plant/Sensor_Model/Sensor_MAG/Magnetometer/Physical_Model/magnetic_field ==
  magnitude_uT : Inport
  declination_deg : Inport  Port=2
  inclination_deg : Inport  Port=3
  Constant : Constant  Value=[1;0;0]  OutDataTypeStr=single
  Gain : Gain  Gain=-pi/180
  Gain1 : Gain  Gain=pi/180
  Multiply : Product
  Multiply1 : Product  Multiplication=Matrix(*)
  Multiply2 : Product  Multiplication=Matrix(*)
  Rotation Matrix Y : FMT_Model_Lib/Transformation/Rotation Matrix Y
      settings: SourceProductName=FMT Toolbox
  Rotation Matrix Z : FMT_Model_Lib/Transformation/Rotation Matrix Z
      settings: SourceProductName=FMT Toolbox
  toGauss : Gain  Gain=0.01
  mag_O_gauss : Outport
  wires:
  Constant/1 -> Multiply/2
  Multiply/1 -> Multiply1/2  "mag_field"
  Rotation Matrix Y/1 -> Multiply1/1
  inclination_deg/1 -> Gain/1
  Gain/1 -> Rotation Matrix Y/1
  declination_deg/1 -> Gain1/1
  Gain1/1 -> Rotation Matrix Z/1
  Rotation Matrix Z/1 -> Multiply2/1
  magnitude_uT/1 -> toGauss/1
  toGauss/1 -> Multiply/1  "magnitude_gauss"
  Multiply1/1 -> Multiply2/2
  Multiply2/1 -> mag_O_gauss/1

== system Plant/Sensor_Model/Sensor_MAG/Magnetometer/Sensor_Model/Sensor_Error ==
  u : Inport
  Add : Sum  InputSameDT=on  OutDataTypeStr=Inherit: Same as first input
  Constant : Constant  Value=eye(3)  OutDataTypeStr=single
  Constant1 : Constant  Value=Sensor_Model.Mag.Scalefactor_Error  VectorParams1D=off  OutDataTypeStr=single
  Constant3 : Constant  Value=Sensor_Model.Mag.Bias  VectorParams1D=off  OutDataTypeStr=single
  Product : Product  Multiplication=Matrix(*)  RndMeth=Zero  InputSameDT=on  OutDataTypeStr=Inherit: Same as first input
  Sum : Sum  Inputs=|++  InputSameDT=on  OutDataTypeStr=Inherit: Same as first input
  y : Outport
  wires:
  Sum/1 -> y/1
  Constant/1 -> Add/1
  Product/1 -> Sum/1
  u/1 -> Product/2
  Constant1/1 -> Add/2
  Add/1 -> Product/1
  Constant3/1 -> Sum/2

== system Plant/Sensor_Model/Sensor_MAG/Magnetometer/Sensor_Model/Sensor_Noise ==
  Random Source : dspsrcs4/Random Source  SrcType=Gaussian  NormMethod=Ziggurat  CltLength=12  MinVal=0  MaxVal=1  MeanVal=0  VarVal=Sensor_Model.Mag.Variance  RepMode=Repeatable  rawSeed=1  IsInherit=off  SampMode=Discrete  SampTime=-1  SampFrame=1  DataType=Single  OutComplex=Real  OutputFrames=off
  noise : Outport
  wires:
  Random Source/1 -> noise/1

== system Plant/Sensor_Model/Sensor_IMU/Accelerometer/Physical_Model/Vibration_Model/vib_frequency ==
  prop_rot_radPs : Inport
  Constant2 : Constant  Value=pi/30*1e4
  Divide2 : Product  Inputs=*/
  u^2 : Math  Operator=square  SaturateOnIntegerOverflow=on
  y : Outport
  wires:
  Divide2/1 -> u^2/1
  prop_rot_radPs/1 -> Divide2/1
  Constant2/1 -> Divide2/2
  u^2/1 -> y/1

== system Plant/Sensor_Model/Sensor_IMU/Gyroscope/Physical_Model/Vibration_Model/vib_frequency ==
  prop_rot_radPs : Inport
  Constant2 : Constant  Value=pi/30*1e4
  Divide2 : Product  Inputs=*/
  u^2 : Math  Operator=square  SaturateOnIntegerOverflow=on
  y : Outport
  wires:
  Divide2/1 -> u^2/1
  prop_rot_radPs/1 -> Divide2/1
  Constant2/1 -> Divide2/2
  u^2/1 -> y/1
